simulink model "mhe_testing"  (R2023b)
settings: Solver=VariableStepAuto  StartTime=0.0  StopTime=500  RelTol=1e-3
values from neighbouring files (symbols this model uses):
  Ts = 0.5    [MHE_compute2.m]
settings Model: Creator=akeebismail  LastModifiedBy=akeebismail

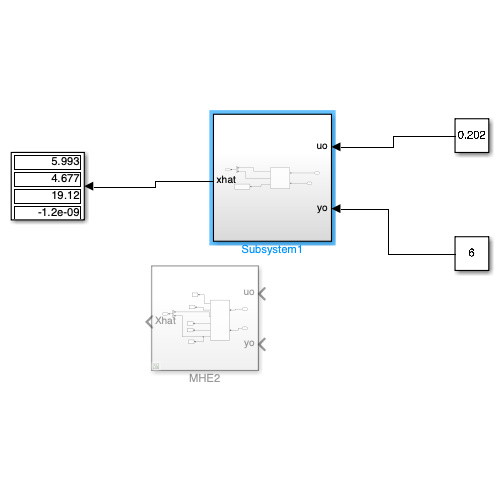
[thumbnail: Simulink's stored preview of the top-level diagram]
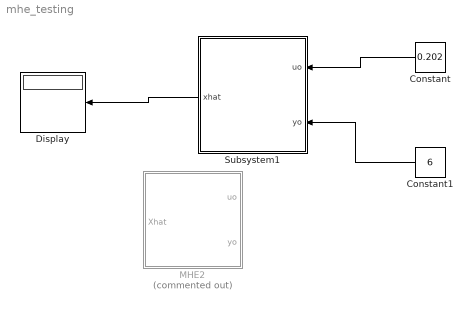
== system mhe_testing ==
  Constant : Constant  Value=0.202
  Constant1 : Constant  Value=6
  Display : Display
  MHE2 : Subsystem  Commented=on
  Subsystem1 : Subsystem
  wires:
  Constant/1 -> Subsystem1/1(uo)
  Constant1/1 -> Subsystem1/2(yo)
  Subsystem1/1(xhat) -> Display/1

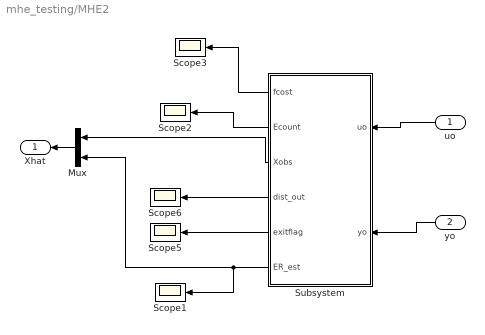
== system mhe_testing/MHE2 ==
  uo : Inport
  yo : Inport  Port=2
  Mux : Mux  Inputs=2
  Scope{1..3,5..6} (5 alike) : Scope
  Subsystem : Subsystem
  Xhat : Outport
  wires:
  Subsystem/3(Xobs) -> Mux/1
  Mux/1 -> Xhat/1
  Subsystem/4(dist_out) -> Scope6/1
  Subsystem/5(exitflag) -> Scope5/1
  Subsystem/6(ER_est) -> Scope1/1, Mux/2
  Subsystem/2(Ecount) -> Scope2/1
  Subsystem/1(fcost) -> Scope3/1
  yo/1 -> Subsystem/2(yo)
  uo/1 -> Subsystem/1(uo)

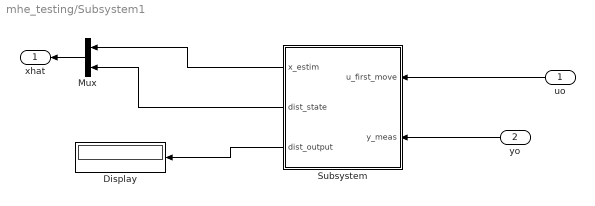
== system mhe_testing/Subsystem1 ==
  uo : Inport
  yo : Inport  Port=2
  Display : Display
  Mux : Mux  Inputs=2
  Subsystem : Subsystem
  xhat : Outport
  wires:
  Mux/1 -> xhat/1
  yo/1 -> Subsystem/2(y_meas)
  uo/1 -> Subsystem/1(u_first_move)
  Subsystem/3(dist_output) -> Display/1
  Subsystem/2(dist_state) -> Mux/2
  Subsystem/1(x_estim) -> Mux/1

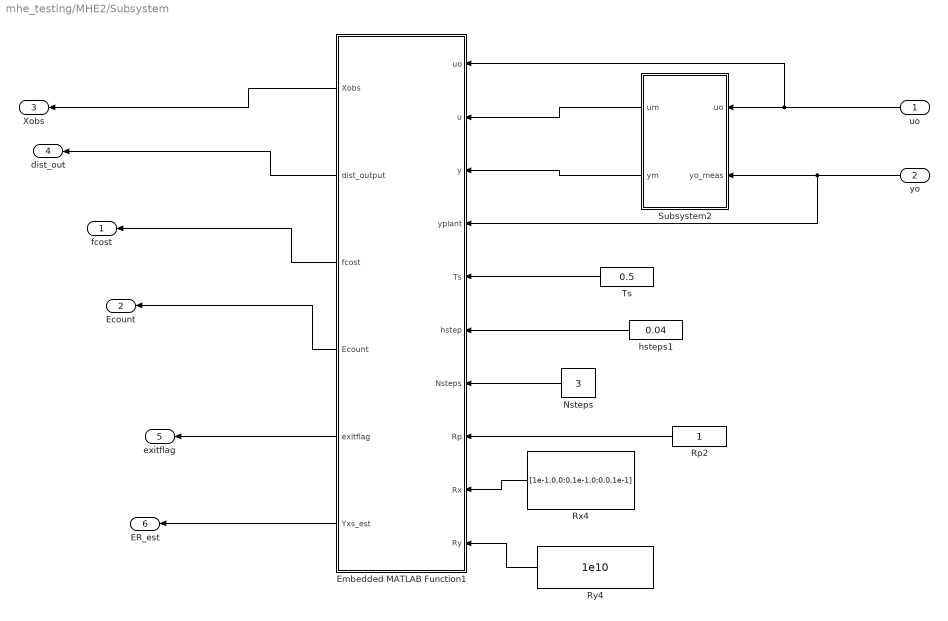
== system mhe_testing/MHE2/Subsystem ==
  uo : Inport
  yo : Inport  Port=2
  Embedded MATLAB Function1 : MATLAB Function  TreatAsAtomicUnit=on
  Nsteps : Constant  Value=3
  Rp2 : Constant
  Rx4 : Constant  Value=[1e-1,0,0;0,1e-1,0;0,0,1e-1]
  Ry4 : Constant  Value=1e10
  Subsystem2 : Subsystem
  Ts : Constant  Value=0.5
  hsteps1 : Constant  Value=0.04
  fcost : Outport  VectorParamsAs1DForOutWhenUnconnected=off
  Ecount : Outport  Port=2  VectorParamsAs1DForOutWhenUnconnected=off
  Xobs : Outport  Port=3  VectorParamsAs1DForOutWhenUnconnected=off
  dist_out : Outport  Port=4  VectorParamsAs1DForOutWhenUnconnected=off
  exitflag : Outport  Port=5  VectorParamsAs1DForOutWhenUnconnected=off
  ER_est : Outport  Port=6  VectorParamsAs1DForOutWhenUnconnected=off
  wires:
  Ts/1 -> Embedded MATLAB Function1/5(Ts)
  Embedded MATLAB Function1/6(Yxs_est) -> ER_est/1
  Embedded MATLAB Function1/5(exitflag) -> exitflag/1
  Embedded MATLAB Function1/2(dist_output) -> dist_out/1
  Embedded MATLAB Function1/1(Xobs) -> Xobs/1
  Ry4/1 -> Embedded MATLAB Function1/10(Ry)
  Rx4/1 -> Embedded MATLAB Function1/9(Rx)
  Rp2/1 -> Embedded MATLAB Function1/8(Rp)
  Embedded MATLAB Function1/4(Ecount) -> Ecount/1
  Embedded MATLAB Function1/3(fcost) -> fcost/1
  hsteps1/1 -> Embedded MATLAB Function1/6(hstep)
  Nsteps/1 -> Embedded MATLAB Function1/7(Nsteps)
  uo/1 -> Subsystem2/1(uo), Embedded MATLAB Function1/1(uo)
  yo/1 -> Subsystem2/2(yo_meas), Embedded MATLAB Function1/4(yplant)
  Subsystem2/2(ym) -> Embedded MATLAB Function1/3(y)
  Subsystem2/1(um) -> Embedded MATLAB Function1/2(u)

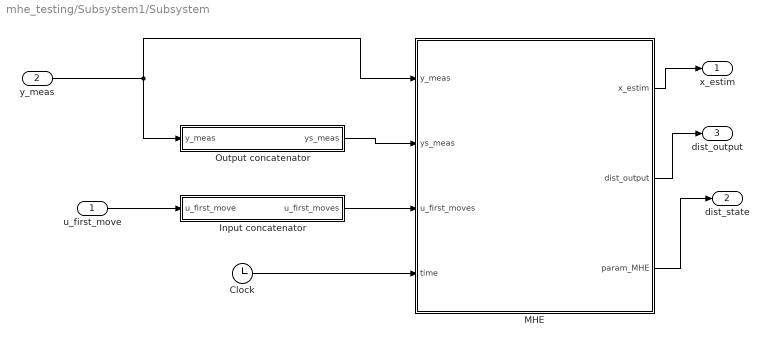
== system mhe_testing/Subsystem1/Subsystem ==
  u_first_move : Inport  PortDimensions=[1,1]
  y_meas : Inport  Port=2  PortDimensions=[1,1]
  Clock : Clock
      settings: Decimation=20
  Input concatenator : Subsystem
  MHE : MATLAB Function  TreatAsAtomicUnit=on
  Output concatenator : Subsystem
  x_estim : Outport
  dist_state : Outport  Port=2
  dist_output : Outport  Port=3
  wires:
  Output concatenator/1(ys_meas) -> MHE/2(ys_meas)
  y_meas/1 -> Output concatenator/1(y_meas), MHE/1(y_meas)
  MHE/1(x_estim) -> x_estim/1
  u_first_move/1 -> Input concatenator/1(u_first_move)
  Clock/1 -> MHE/4(time)
  MHE/2(dist_output) -> dist_output/1
  MHE/3(param_MHE) -> dist_state/1
  Input concatenator/1(u_first_moves) -> MHE/3(u_first_moves)

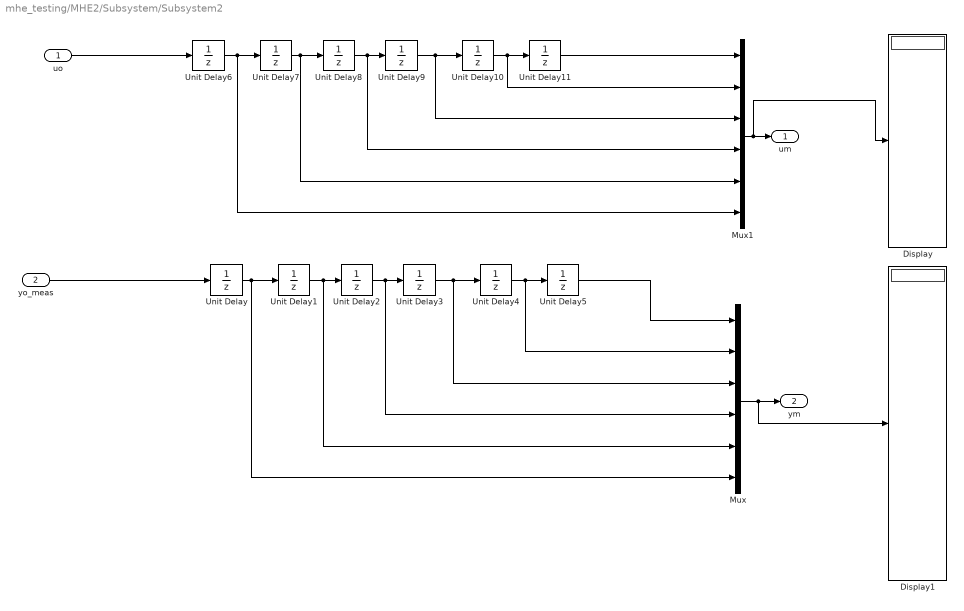
== system mhe_testing/MHE2/Subsystem/Subsystem2 ==
  uo : Inport
  yo_meas : Inport  Port=2
  Display : Display
  Display1 : Display
  Mux : Mux  Inputs=6
  Mux1 : Mux  Inputs=6
  Unit Delay{,1..5} (6 alike) : UnitDelay  InitialCondition=6  SampleTime=Ts  HasFrameUpgradeWarning=on
  Unit Delay{6..11} (6 alike) : UnitDelay  InitialCondition=0.202  SampleTime=Ts  HasFrameUpgradeWarning=on
  um : Outport  VectorParamsAs1DForOutWhenUnconnected=off
  ym : Outport  Port=2  VectorParamsAs1DForOutWhenUnconnected=off
  wires:
  yo_meas/1 -> Unit Delay/1
  Unit Delay5/1 -> Mux/1
  Unit Delay11/1 -> Mux1/1
  Mux1/1 -> Display/1, um/1
  Mux/1 -> Display1/1, ym/1
  Unit Delay10/1 -> Mux1/2, Unit Delay11/1
  Unit Delay9/1 -> Unit Delay10/1, Mux1/3
  Unit Delay8/1 -> Unit Delay9/1, Mux1/4
  Unit Delay7/1 -> Unit Delay8/1, Mux1/5
  Unit Delay6/1 -> Unit Delay7/1, Mux1/6
  uo/1 -> Unit Delay6/1
  Unit Delay4/1 -> Mux/2, Unit Delay5/1
  Unit Delay3/1 -> Mux/3, Unit Delay4/1
  Unit Delay2/1 -> Mux/4, Unit Delay3/1
  Unit Delay1/1 -> Mux/5, Unit Delay2/1
  Unit Delay/1 -> Mux/6, Unit Delay1/1

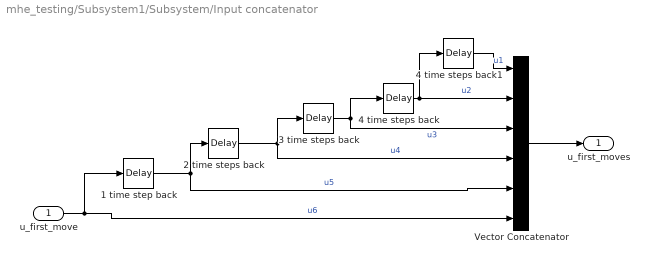
== system mhe_testing/Subsystem1/Subsystem/Input concatenator ==
  u_first_move : Inport
  1 time step back : TransportDelay  DelayTime=Ts  InitialOutput=0.202
  2 time steps back : TransportDelay  DelayTime=Ts  InitialOutput=0.202
  3 time steps back : TransportDelay  DelayTime=Ts  InitialOutput=0.202
  4 time steps back : TransportDelay  DelayTime=Ts  InitialOutput=0.202
  4 time steps back1 : TransportDelay  DelayTime=Ts  InitialOutput=0.202
  Vector Concatenator : Concatenate  NumInputs=6  Mode=Multidimensional array
  u_first_moves : Outport  PortDimensions=[6,1]  VectorParamsAs1DForOutWhenUnconnected=off
  wires:
  4 time steps back1/1 -> Vector Concatenator/1  "u1"
  1 time step back/1 -> Vector Concatenator/5, 2 time steps back/1  "u5"
  2 time steps back/1 -> Vector Concatenator/4, 3 time steps back/1  "u4"
  3 time steps back/1 -> 4 time steps back/1, Vector Concatenator/3  "u3"
  4 time steps back/1 -> 4 time steps back1/1, Vector Concatenator/2  "u2"
  u_first_move/1 -> 1 time step back/1, Vector Concatenator/6  "u6"
  Vector Concatenator/1 -> u_first_moves/1

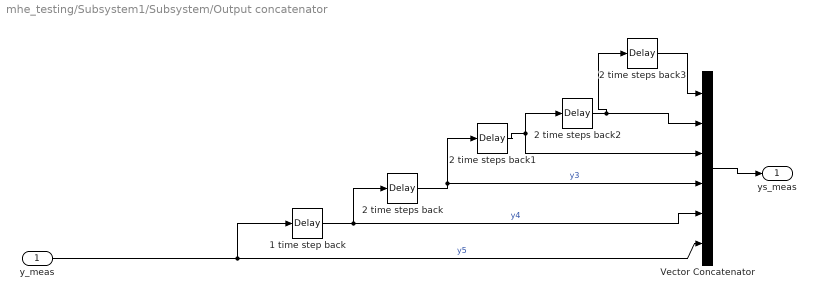
== system mhe_testing/Subsystem1/Subsystem/Output concatenator ==
  y_meas : Inport
  1 time step back : TransportDelay  DelayTime=Ts  InitialOutput=6
  2 time steps back{,1..3} (4 alike) : TransportDelay  DelayTime=Ts  InitialOutput=6
  Vector Concatenator : Concatenate  NumInputs=6  Mode=Multidimensional array
  ys_meas : Outport  PortDimensions=[6,1]  VectorParamsAs1DForOutWhenUnconnected=off
  wires:
  2 time steps back3/1 -> Vector Concatenator/1
  y_meas/1 -> 1 time step back/1, Vector Concatenator/6  "y5"
  1 time step back/1 -> 2 time steps back/1, Vector Concatenator/5  "y4"
  2 time steps back/1 -> Vector Concatenator/4, 2 time steps back1/1  "y3"
  Vector Concatenator/1 -> ys_meas/1
  2 time steps back1/1 -> Vector Concatenator/3, 2 time steps back2/1
  2 time steps back2/1 -> Vector Concatenator/2, 2 time steps back3/1

== matlab function mhe_testing/Subsystem1/Subsystem/MHE ==
  data: y_meas input; ys_meas input; x_estim output; u_first_moves input; time input; dist_output output; param_MHE output
function [x_estim,dist_output,param_MHE] = MHE_4_tanks(y_meas,ys_meas,u_first_moves,time)

coder.extrinsic('MHE_compute2');

N_MHE=6  ;
% Ts=2 ;


if time < 5
    
    x_estim =  [6;5;19.14]  ;
   % x_estim = [17;17;17];
    %x_estim = [5.898;1.8];
    param_MHE = 0.4;
    dist_output = 0;
else
    
    [x_estim,param_MHE,dist_output] = MHE_compute2(ys_meas,u_first_moves,N_MHE,y_meas);
    %Note that our horizon must be constant here. It is chosen as 5.
end

end

== matlab function mhe_testing/MHE2/Subsystem/Embedded MATLAB Function1 ==
  data: uo input; Xobs output size=[3,1]; dist_output output size=[1,1]; u input; y input; yplant input; Ts input; hstep input; Nsteps input; Rp input; fcost output size=[1,1]; Rx input; Ry input; Ecount output size=[1,1]; exitflag output size=[1,1]; Yxs_est output size=[1,1]
function [Xobs,dist_output,fcost,Ecount,exitflag,Yxs_est] =MHE(uo,u,y,yplant,Ts,hstep,Nsteps,Rp,Rx,Ry)

%#codegen
coder.extrinsic('MHE_compute','clear_var');

um=[u(1),u(2),u(3),u(4),u(5),u(6)] ;
 

ymeas=[y(1),y(2),y(3),y(4),y(5),y(6)] ;


    
   

% SAMPLING TIME FOR DISCRETIZATION
%hstep=1; %sampling time of 10 is with less interation while 5 is smoother but higher interaction
%Nsteps=1 ;% Nsteps=10 ; % Nsteps=20 ;


d_initial=[6;5;19.14;0.4]   ;
%d_MIN_colvector =[0;0;100]  ;
d_MIN_colvector =[0;0;0;0]  ;
d_MAX_colvector =[20;60;60;1]  ;
%%%%%%%%%%%%%%%%%%%%%%%%%%%%%%%%%%%%%%%
%Initializing variables
fcost=inf  ;
Xobs=[0;0;0]  ;
%d_opt=[0;0]  ;
dist_output = [0]  ;
Yxs_est=[0]  ;
Ecount=0  ;
exitflag=2   ;

% [Xobs,dist_output,fcost,Ecount,exitflag]=MHE_compute(uo,um,ymeas,yplant...
%                                         ,hstep,Nsteps,Nmhe,Rp,Rx,Ry...
%                                         ,p_initial, p_MIN_colvector,p_MAX_colvector)
[Xobs,dist_output,Yxs_est,fcost,Ecount,exitflag]=MHE_compute(uo,um,ymeas...
                                        ,yplant,Ts,hstep,Nsteps,Rp,Rx,Ry...
                                        ,d_initial, d_MIN_colvector,d_MAX_colvector);
